simulink subsystem "encoder"  (R2022b)
settings: Solver=VariableStepAuto  StartTime=0.0  StopTime=10.0  RelTol=1e-3
settings Model: Creator=LeonK  LastModifiedBy=LeonK

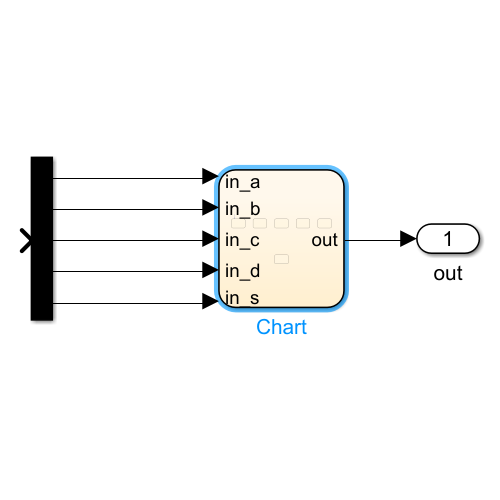
[thumbnail: Simulink's stored preview of the top-level diagram]
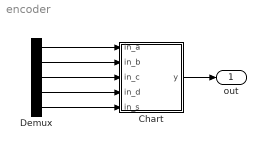
== system encoder ==
  Chart : Stateflow chart  TreatAsAtomicUnit=on
  Demux : Demux  Outputs=5
  out : Outport
  wires:
  Demux/1 -> Chart/1(in_a)
  Demux/2 -> Chart/2(in_b)
  Demux/3 -> Chart/3(in_c)
  Demux/4 -> Chart/4(in_d)
  Demux/5 -> Chart/5(in_s)
  Chart/1(y) -> out/1

== stateflow chart encoder/Chart ==
  state q_initialize
  state q_0_10
  state q_10_20
  state q_20_30
  state q_30_max
  state flooding
  state q_malfunction
  q_initialize -> q_30_max [order 2] : [in_a==1]{y=1}
  q_0_10 -> q_10_20 [order 1] : [in_c==1]{y=1}
  (default) -> q_initialize
  q_initialize -> q_0_10 [order 1] : [in_d==0]{y=0}
  q_10_20 -> q_20_30 [order 1] : [in_b==1]{y=1}
  q_20_30 -> q_30_max [order 1] : [in_a==1]{y=1}
  q_30_max -> flooding [order 2] : [in_s==1]{y=0000}
  q_0_10 -> q_malfunction [order 2]
  q_10_20 -> q_0_10 [order 2] : [in_a==0]{y=0}
  q_10_20 -> q_malfunction [order 3]
  q_20_30 -> q_10_20 [order 2] : [in_b==0]{y=0}
  q_20_30 -> q_malfunction [order 3]
  q_30_max -> q_malfunction [order 3]
  q_30_max -> q_20_30 [order 1] : [in_a==0]{y=0}
  flooding -> q_malfunction
  data: in_a input; in_b input; in_c input; in_d input; in_s input; y output
